simulink model "Registro"  (R2020a)
settings: Solver=VariableStepAuto  StartTime=0.0  StopTime=40  RelTol=1e-3
settings Model: DataDictionary=Registro_variables.sldd  Creator=Juan  LastModifiedBy=Juan

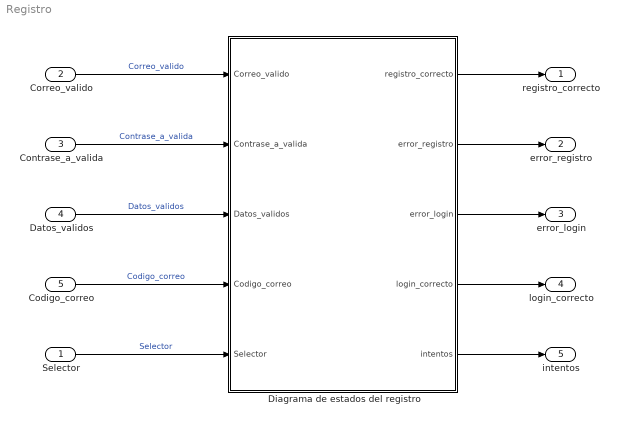
== system Registro ==
  Selector : Inport  OutMin=0  OutMax=2  OutDataTypeStr=double  PortDimensions=1
  Correo_valido : Inport  Port=2  OutMin=0  OutMax=1  OutDataTypeStr=boolean  PortDimensions=1
  Contrase_a_valida : Inport  Port=3  OutMin=0  OutMax=1  OutDataTypeStr=boolean  PortDimensions=1
  Datos_validos : Inport  Port=4  OutMin=0  OutMax=1  OutDataTypeStr=boolean  PortDimensions=1
  Codigo_correo : Inport  Port=5  OutMin=0  OutMax=1  OutDataTypeStr=boolean  PortDimensions=1
  Diagrama de estados del registro : Stateflow chart  TreatAsAtomicUnit=on
  registro_correcto : Outport  SignalName=registro_correcto  OutMin=0  OutMax=1  OutDataTypeStr=boolean  PortDimensions=1  VectorParamsAs1DForOutWhenUnconnected=off
      settings: MustResolveToSignalObject=on
  error_registro : Outport  Port=2  SignalName=error_registro  OutMin=0  OutMax=1  OutDataTypeStr=boolean  PortDimensions=1  VectorParamsAs1DForOutWhenUnconnected=off
      settings: MustResolveToSignalObject=on
  error_login : Outport  Port=3  SignalName=error_login  OutMin=0  OutMax=1  OutDataTypeStr=boolean  PortDimensions=1  VectorParamsAs1DForOutWhenUnconnected=off
      settings: MustResolveToSignalObject=on
  login_correcto : Outport  Port=4  SignalName=login_correcto  OutMin=0  OutMax=1  OutDataTypeStr=boolean  PortDimensions=1  VectorParamsAs1DForOutWhenUnconnected=off
      settings: MustResolveToSignalObject=on
  intentos : Outport  Port=5  SignalName=intentos  OutMin=0  OutMax=30  OutDataTypeStr=double  PortDimensions=1  VectorParamsAs1DForOutWhenUnconnected=off
      settings: MustResolveToSignalObject=on
  wires:
  Contrase_a_valida/1 -> Diagrama de estados del registro/2(Contrase_a_valida)  "Contrase_a_valida"
  Datos_validos/1 -> Diagrama de estados del registro/3(Datos_validos)  "Datos_validos"
  Codigo_correo/1 -> Diagrama de estados del registro/4(Codigo_correo)  "Codigo_correo"
  Diagrama de estados del registro/1(registro_correcto) -> registro_correcto/1
  Correo_valido/1 -> Diagrama de estados del registro/1(Correo_valido)  "Correo_valido"
  Selector/1 -> Diagrama de estados del registro/5(Selector)  "Selector"
  Diagrama de estados del registro/2(error_registro) -> error_registro/1
  Diagrama de estados del registro/3(error_login) -> error_login/1
  Diagrama de estados del registro/4(login_correcto) -> login_correcto/1
  Diagrama de estados del registro/5(intentos) -> intentos/1

== stateflow chart Registro/Diagrama de estados del registro ==
  state OFF
    error_login=false
    error_registro = false
    intentos = 0
    login_correcto = false
  state ERROR_LOGIN
    error_login = true
  state ERROR_REGISTRO
    error_registro = true
  state REGISTRO
    state INTRODUCIR_CORREO
      registro_correcto = false
      intentos = intentos + 1
    state REGISTRO_CORRECTO
      registro_correcto = true
    state INTRODUCIR_CONTRASE_A
      registro_correcto = false
      intentos = intentos + 1
    state ENVIAR_CORREO
      intentos = ++intentos
    state INTRODUCIR_OTROS_DATOS
      registro_correcto = false
      intentos = intentos + 1
    state VERIFICACION_DOS_PASOS
      registro_correcto = false
    (default) -> REGISTRO.INTRODUCIR_CORREO
    REGISTRO.INTRODUCIR_CORREO -> REGISTRO.INTRODUCIR_CORREO [order 2] : [~Correo_valido && intentos <= 100]
    REGISTRO.INTRODUCIR_CORREO -> REGISTRO.INTRODUCIR_CONTRASE_A [order 1] : [Correo_valido && intentos <= 100]
    REGISTRO.INTRODUCIR_CONTRASE_A -> REGISTRO.INTRODUCIR_CONTRASE_A [order 1] : [~Contrase_a_valida && intentos <=100]
    REGISTRO.ENVIAR_CORREO -> REGISTRO_CORRECTO [order 1] : [Codigo_correo && intentos<=200]
    REGISTRO.ENVIAR_CORREO -> REGISTRO.ENVIAR_CORREO [order 3] : [~Codigo_correo]
    REGISTRO.VERIFICACION_DOS_PASOS -> REGISTRO.ENVIAR_CORREO : [~Codigo_correo && intentos<=200]
    REGISTRO.INTRODUCIR_CONTRASE_A -> INTRODUCIR_OTROS_DATOS [order 2] : [Contrase_a_valida && intentos<=100]
    INTRODUCIR_OTROS_DATOS -> INTRODUCIR_OTROS_DATOS [order 1] : [~Datos_validos && intentos<=200]
    INTRODUCIR_OTROS_DATOS -> REGISTRO.VERIFICACION_DOS_PASOS [order 2] : [Datos_validos && intentos<=200]
  state LOGIN
    en:
    intentos = 0
    state LOGIN_CORRECTO
      login_correcto = true
    state INTRODUCIR_CORREO
      intentos = ++intentos
      login_correcto = false
      registro_correcto = false
    state ENVIAR_CORREO
      intentos = ++intentos
    state INTRODUCIR_CONTRASE_A
      login_correcto = false
      intentos = ++intentos
    state VERIFICACION_DOS_PASOS
      login_correcto = false
    (default) -> LOGIN.INTRODUCIR_CORREO
    LOGIN.ENVIAR_CORREO -> LOGIN_CORRECTO [order 3] : [Codigo_correo && intentos<=200]
    LOGIN.INTRODUCIR_CORREO -> LOGIN.INTRODUCIR_CORREO [order 1] : [~Correo_valido && intentos <= 200]
    LOGIN.ENVIAR_CORREO -> LOGIN.ENVIAR_CORREO [order 1] : [~Codigo_correo]
    LOGIN.INTRODUCIR_CORREO -> LOGIN.INTRODUCIR_CONTRASE_A [order 2] : [Correo_valido && intentos <= 200]
    LOGIN.VERIFICACION_DOS_PASOS -> LOGIN.ENVIAR_CORREO : [~Codigo_correo && intentos<=200]
    LOGIN.INTRODUCIR_CONTRASE_A -> LOGIN.INTRODUCIR_CONTRASE_A [order 1] : [~Contrase_a_valida && intentos<=500]
    LOGIN.INTRODUCIR_CONTRASE_A -> LOGIN.VERIFICACION_DOS_PASOS [order 3] : [Contrase_a_valida && intentos<=200]
  (default) -> OFF
  LOGIN_CORRECTO -> OFF : [login_correcto]
  OFF -> REGISTRO [order 1] : [Selector==1]
  OFF -> OFF [order 3] : [Selector==0]
  LOGIN.ENVIAR_CORREO -> ERROR_LOGIN [order 2] : [intentos>200]
  LOGIN.INTRODUCIR_CONTRASE_A -> ERROR_LOGIN [order 2] : [intentos>200]
  REGISTRO_CORRECTO -> OFF : [registro_correcto]
  OFF -> LOGIN [order 2] : [Selector == 2]
  REGISTRO.ENVIAR_CORREO -> ERROR_REGISTRO [order 2] : [intentos>100]
  LOGIN.INTRODUCIR_CORREO -> ERROR_LOGIN [order 3] : [intentos>200]
  INTRODUCIR_OTROS_DATOS -> ERROR_REGISTRO [order 3] : [intentos>200]
  REGISTRO.INTRODUCIR_CONTRASE_A -> ERROR_REGISTRO [order 3] : [intentos>100]
  REGISTRO.INTRODUCIR_CORREO -> ERROR_REGISTRO [order 3] : [intentos > 100]
  data: Correo_valido input; Contrase_a_valida input; Datos_validos input; Codigo_correo input; registro_correcto output; Selector input; error_registro output; error_login output; login_correcto output; intentos output int64
